simulink model "Conditionalbasic"  (R2022a)
settings: Solver=VariableStepAuto  StartTime=0.0  StopTime=inf  RelTol=1e-3
libraries: simulink x1
settings Model: Creator=JWilliams_E_E  LastModifiedBy=JWilliams_E_E

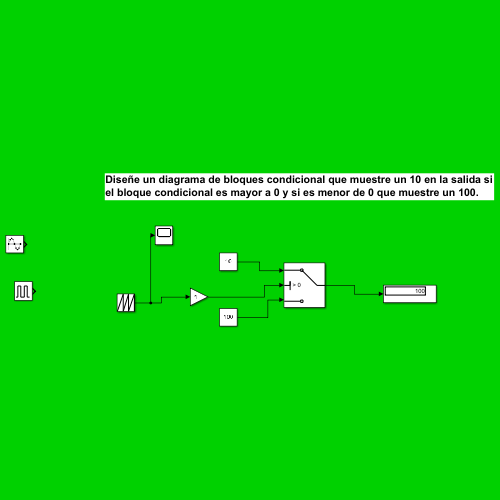
[thumbnail: Simulink's stored preview of the top-level diagram]
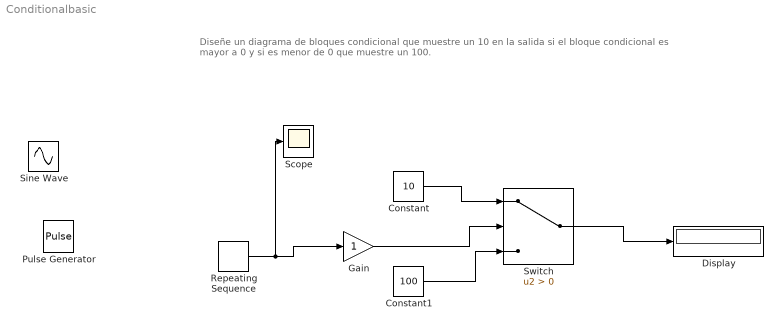
== system Conditionalbasic ==
  note: Diseñe un diagrama de bloques condicional que muestre un 10 en la salida si el bloque condicional es mayor a 0 y si es menor de 0 que muestre un 100.
  Constant : Constant  Value=10
  Constant1 : Constant  Value=100
  Display : Display
  Gain : Gain
  Pulse Generator : DiscretePulseGenerator  PulseType=Time based  Period=1  PulseWidth=50
  Repeating Sequence : simulink/Sources/Repeating Sequence  rep_seq_t=[-1 1]  rep_seq_y=[-2 2]
  Scope : Scope
  Sine Wave : Sin  SineType=Sample based  Samples=5  SampleTime=5e-6
  Switch : Switch  Criteria=u2 > Threshold  SaturateOnIntegerOverflow=off  InputSameDT=off
  wires:
  Switch/1 -> Display/1
  Gain/1 -> Switch/2
  Repeating Sequence/1 -> Scope/1, Gain/1
  Constant/1 -> Switch/1
  Constant1/1 -> Switch/3
